simulink model "test_template_sim"  (R2022b)
settings: Solver=FixedStepAuto  StartTime=0.0  StopTime=inf  RelTol=1e-3
libraries: arduinosensorlib x1, arduinolib x1
settings Model: ExtModeTrigDuration=2  Creator=shantamerkanian  LastModifiedBy=shantamerkanian
settings OptimizationCC: EnhancedBackFolding=on  PassReuseOutputArgsAs=Individual arguments  ZeroExternalMemoryAtStartup=off  ZeroInternalMemoryAtStartup=off  MaxStackSize=64  OptimizeBlockOrder=speed  DifferentSizesBufferReuse=on  OptimizationCustomize=off  EfficientTunableParamExpr=on
settings DebuggingCC: ParameterTunabilityLossMsg=error
settings HardwareCC: ProdBitPerInt=16  ProdBitPerPointer=16  ProdBitPerSizeT=16  ProdBitPerPtrDiffT=16  ProdLargestAtomicFloat=None  ProdWordSize=8  ProdHWDeviceType=Atmel->AVR  UseEmbeddedCoderFeatures=off  UseSimulinkCoderFeatures=off
settings SFSimCC: MATLABDynamicMemAlloc=off
settings RTWCC: Description=Embedded Coder  SystemTargetFile=ert.tlc  HardwareBoard=Arduino Mega 2560  TLCOptions=-aInlineSetEventsForThisBaseRateFcn=TLC_FALSE -aSuppressMultiTaskScheduler=TLC_FALSE -aRateBasedStepFcn=1  TemplateMakefile=ert_default_tmf  Toolchain=Arduino AVR
settings CodeAppCC: ForceParamTrailComments=on  IgnoreCustomStorageClasses=off  OperatorAnnotations=on  SimulinkDataObjDesc=on  SFDataObjDesc=on  MangleLength=10  InsertBlockDesc=on
settings ERTTargetCC: SupportContinuousTime=on  SupportNonInlinedSFcns=on  SupportVariableSizeSignals=on  ExtModeTransport=3  ExtModeStaticAlloc=on  ExtModeAutomaticAllocSize=off  ExtModeStaticAllocSize=2048  ExtModeMexFile=ext_xcp  ExtModeIntrfLevel=Level2 - Open

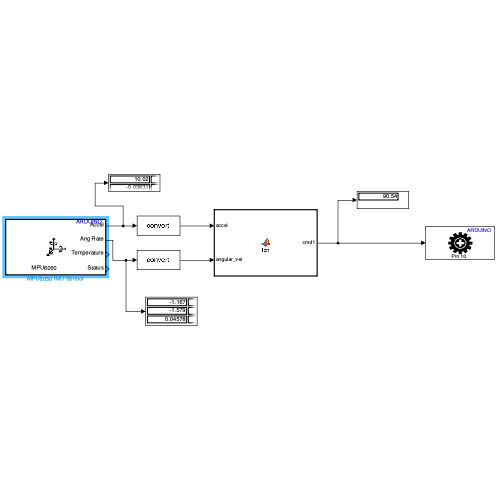
[thumbnail: Simulink's stored preview of the top-level diagram]
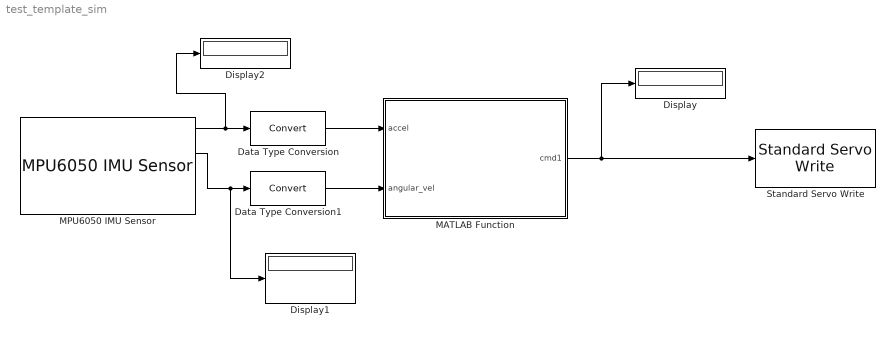
== system test_template_sim ==
  Data Type Conversion : DataTypeConversion  SaturateOnIntegerOverflow=off  RndMeth=Floor
  Data Type Conversion1 : DataTypeConversion  SaturateOnIntegerOverflow=off  RndMeth=Floor
  Display : Display
  Display1 : Display
  Display2 : Display
  MATLAB Function : MATLAB Function  TreatAsAtomicUnit=on
  MPU6050 IMU Sensor : arduinosensorlib/MPU6050 IMU Sensor  SlaveAddress=0x68  Accel=on  AngularRate=on  Temperature=on  Status=on  Timestamp=off  EulerAngles=off  Quat=off  AccelRange=2G  GyroRange=250 dps  DmpOdr=200 Hz  Dlpf=Accelerometer: 184Hz, Gyroscope: 188Hz  spf=4  SampleTime=.004  QueueSizeFactor=4
  Standard Servo Write : arduinolib/Standard Servo Write  pinNumber=10  ServoIndex=0  blockPlatform=ARDUINO
  wires:
  MPU6050 IMU Sensor/1 -> Display2/1, Data Type Conversion/1
  MPU6050 IMU Sensor/2 -> Display1/1, Data Type Conversion1/1
  MATLAB Function/1(cmd1) -> Standard Servo Write/1, Display/1
  Data Type Conversion/1 -> MATLAB Function/1(accel)
  Data Type Conversion1/1 -> MATLAB Function/2(angular_vel)

== matlab function test_template_sim/MATLAB Function ==
  data: cmd1 output; accel input; angular_vel input
function cmd1  = fcn(accel,  angular_vel)
    % Start timer to check duration of control loop
    Kd = [2.21 2.89];
    
    % Read IMU and Calculate State
    imu_offset = .01;
    g = 9.8066;

    % Read
    a_x = accel(1);
    a_y = accel(2);
    a_z = accel(3);
    p = angular_vel(1);
    q = angular_vel(2);
    r = angular_vel(3);

    % Calcualte adjusted acceleration TODO: choose different based on
    % orientation
    radial = p^2*imu_offset;
    a_y = a_y - radial;
    theta = asind(a_y/g);

    % Write current values to the SD card (or outsource to DAS arduino)
    
    xp = [theta; r]; % Plant state
    % Currently: unknown orientation of IMU in housing, structure
    % should be correct

    % Calculate desired servo value
    u = -Kd*xp;
    if abs(u) > 15
        u = (abs(u)/u)*15;
    end
    cmd1 = 90+u;

end
